simulink model "simulink_implementation"  (R2021b)
settings: Solver=FixedStepDiscrete  StartTime=0.0  StopTime=10  FixedStep=0.02  RelTol=1e-3
values from neighbouring files (symbols this model uses):
  constraint = struct()    [bicycle_model.m]
  model = struct()    [bicycle_model.m]
  N = 50    [main.m]
settings Model: PauseTimes=0.4  Creator=KURAPAS  LastModifiedBy=KURAPAS

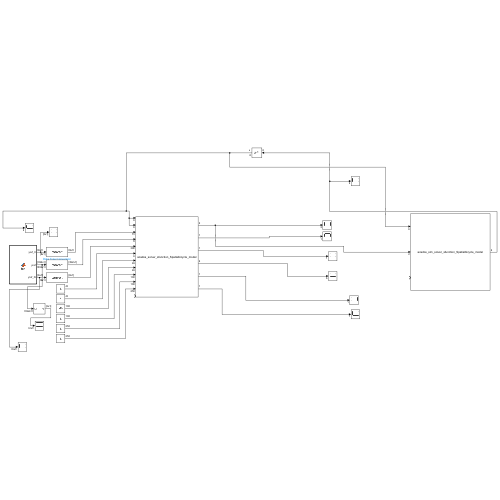
[thumbnail: Simulink's stored preview of the top-level diagram]
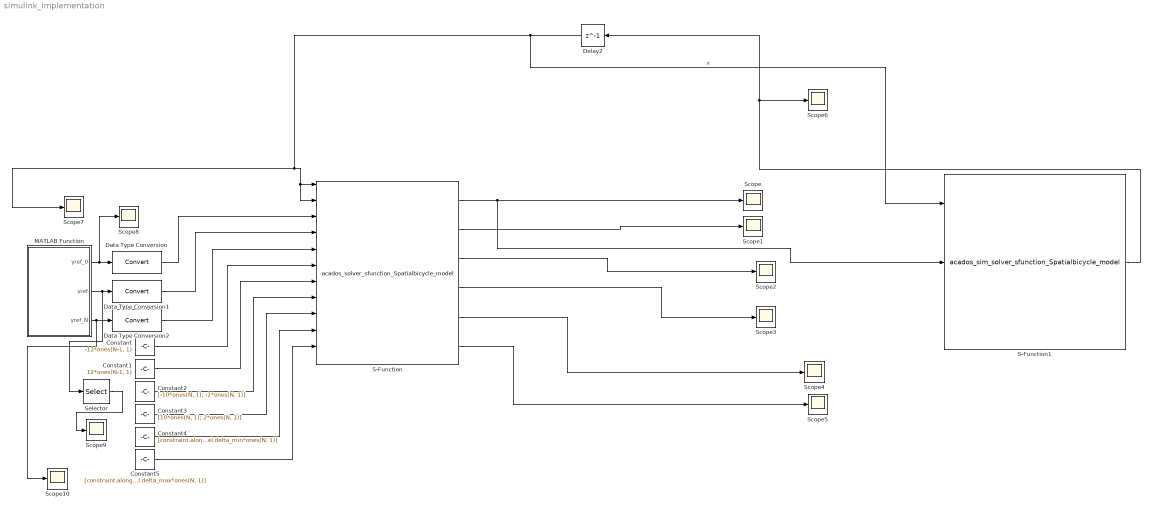
== system simulink_implementation ==
  Constant : Constant  Value=-12*ones(N-1, 1)
  Constant1 : Constant  Value=12*ones(N-1, 1)
  Constant2 : Constant  Value=[-10*ones(N, 1); -2*ones(N, 1)]
  Constant3 : Constant  Value=[10*ones(N, 1); 2*ones(N, 1)]
  Constant4 : Constant  Value=[constraint.along_min*ones(N, 1);constraint.alat_min*ones(N, 1);model.n_min*ones(N, 1);model.throttle_min*ones(N, 1);model.delta_min*ones(N, 1)]
  Constant5 : Constant  Value=[constraint.along_max*ones(N, 1);constraint.alat_max*ones(N, 1);model.n_max*ones(N, 1);model.throttle_max*ones(N, 1);model.delta_max*ones(N, 1)]
  Data Type Conversion : DataTypeConversion
  Data Type Conversion1 : DataTypeConversion
  Data Type Conversion2 : DataTypeConversion
  Delay2 : Delay  DelayLength=1  InitialCondition=[-2;0;0;0;0;0]
  MATLAB Function : MATLAB Function  TreatAsAtomicUnit=on
  S-Function : S-Function  FunctionName=acados_solver_sfunction_Spatialbicycle_model  SFunctionDeploymentMode=off  EnableBusSupport=off
  S-Function1 : S-Function  FunctionName=acados_sim_solver_sfunction_Spatialbicycle_model  SFunctionDeploymentMode=off  EnableBusSupport=off
  Scope{,1..10} (11 alike) : Scope
  Selector : Selector  IndexOptions=Index vector (dialog)  Indices=[1 1]  OutputSizes=1
  wires:
  S-Function1/1 -> Scope6/1, Delay2/1
  Delay2/1 -> S-Function1/1, Scope7/1, S-Function/2, S-Function/1  "x"
  S-Function/1 -> S-Function1/2, Scope/1
  S-Function/2 -> Scope1/1
  S-Function/3 -> Scope2/1
  S-Function/4 -> Scope3/1
  S-Function/5 -> Scope4/1
  S-Function/6 -> Scope5/1
  MATLAB Function/1(yref_0) -> Scope8/1, Data Type Conversion/1
  MATLAB Function/2(yref) -> Selector/1, Data Type Conversion1/1
  MATLAB Function/3(yref_N) -> Scope10/1, Data Type Conversion2/1
  Data Type Conversion/1 -> S-Function/3
  Data Type Conversion1/1 -> S-Function/4
  Data Type Conversion2/1 -> S-Function/5
  Constant/1 -> S-Function/6
  Constant1/1 -> S-Function/7
  Constant2/1 -> S-Function/8
  Constant3/1 -> S-Function/9
  Constant4/1 -> S-Function/10
  Constant5/1 -> S-Function/11
  Selector/1 -> Scope9/1

== matlab function simulink_implementation/MATLAB Function ==
  data: yref_0 output; yref output; yref_N output
function [yref_0, yref, yref_N] = fcn()
% sref_N =5; 
N =50;
% s0 = x(1);
% yref = zeros(392,1);
% sref = s0 + sref_N;
% if(sim_time<0.2)
%      sref = s0 + sref_N;
%      yref_0 = [s0; 0; 0; 0; 0; 0; 0; 0];
% else
%     sref = s0 +sref_N;
%     yref_0 = [s0; 0; 0; 0; 0; 0; 0; 0];
% end
%  
% for j = 0:N-1
%     yref(j+1) = [s0 + (sref - s0) * j / N];
% end
yref_0 = [1; 0; 0; 0; 0; 0; 0; 0];
yref = repmat(yref_0, N-1, 1)
% yref(:) =[zeros(8*(N-1),1)];
yref_N = [0; 0; 0; 0; 0; 0];

end
